simulink subsystem "ControladorBA"  (R2023b)
settings: Solver=VariableStepAuto  StartTime=0.0  StopTime=10.0  RelTol=1e-3
settings Model: Creator=Claudia Ada  LastModifiedBy=pablo

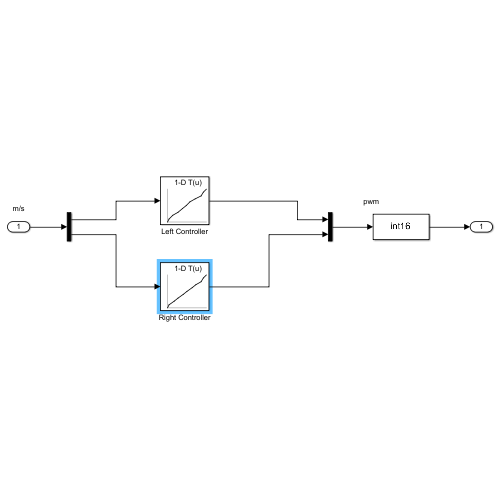
[thumbnail: Simulink's stored preview of the top-level diagram]
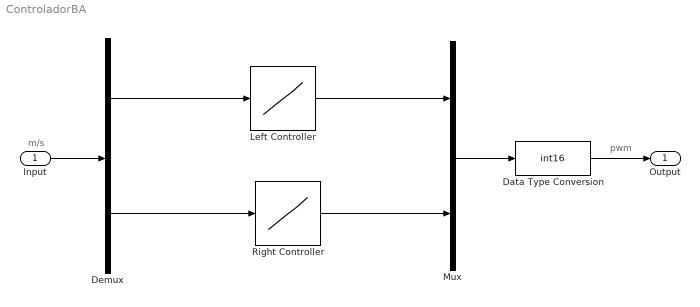
== system ControladorBA ==
  note: pwm
  note: m/s
  Input : Inport
  Data Type Conversion : DataTypeConversion  OutDataTypeStr=int16  SaturateOnIntegerOverflow=off  RndMeth=Floor
  Demux : Demux  Outputs=2
  Left Controller : Lookup_n-D  NumberOfTableDimensions=1  BreakpointsForDimension1=[-0.199222564697266 -0.184992790222168 -0.142301559448242 -0.085381031036377 -0.042690634727478 0 0.042694091796875 0.099609375 0.156532287597656 0.18499755859375 0.213447570800781]  Table=[-100 -80 -60 -40 -20 0 20 40 60 80 100]  InternalRulePriority=Speed  RndMeth=Simplest
  Mux : Mux  Inputs=2
  Right Controller : Lookup_n-D  NumberOfTableDimensions=1  BreakpointsForDimension1=[-0.213452339172363 -0.199223041534424 -0.14230227470398 -0.0996114611625671 -0.042690634727478 0 0.056922912597656 0.099609375 0.156532287597656 0.184989929199219 0.213447570800781]  Table=[-100 -80 -60 -40 -20 0 20 40 60 80 100]  InternalRulePriority=Speed  RndMeth=Simplest
  Output : Outport
  wires:
  Demux/1 -> Left Controller/1
  Left Controller/1 -> Mux/1
  Demux/2 -> Right Controller/1
  Right Controller/1 -> Mux/2
  Input/1 -> Demux/1
  Mux/1 -> Data Type Conversion/1
  Data Type Conversion/1 -> Output/1
